simulink model "test1"  (R2017b)
settings: Solver=VariableStepAuto  StartTime=0.0  StopTime=10.0  RelTol=1e-3
settings Model: Creator=flosch  LastModifiedBy=flosch

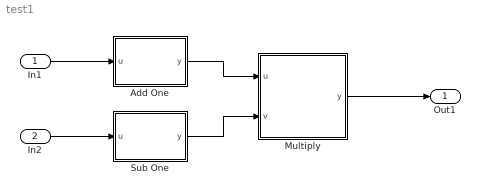
== system test1 ==
  In1 : Inport
  In2 : Inport  Port=2
  Add One : MATLAB Function  TreatAsAtomicUnit=on
  Multiply : MATLAB Function  TreatAsAtomicUnit=on
  Sub One : MATLAB Function  TreatAsAtomicUnit=on
  Out1 : Outport
  wires:
  Add One/1(y) -> Multiply/1(u)
  Sub One/1(y) -> Multiply/2(v)
  In1/1 -> Add One/1(u)
  In2/1 -> Sub One/1(u)
  Multiply/1(y) -> Out1/1

== matlab function test1/Sub One ==
  data: u input; y output
function y = sub_one(u)

y = u - 1;

== matlab function test1/Add One ==
  data: u input; y output
function y = add_one(u)

y = u + 1;

== matlab function test1/Multiply ==
  data: u input; y output; v input
function y = my_multiply(u, v)

y = u * v;
